simulink model "example_RIEKF"  (R2017b)
settings: Solver=FixedStepDiscrete  StartTime=0.0  StopTime=outputs.messages.Time(end)  RelTol=1e-3  EnableMultiTasking=on
InitFcn:
  | CassieModule.importBuses;
undefined symbols (not defined in the file or in its folder): R0, v0
libraries: lib_StateEstimation x7
settings Model: ParamWorkspaceSource=ReferencedWorkspace  Creator=robot  LastModifiedBy=nboyd
settings DataIOCC: SaveFormat=Array  SaveOutput=off  SignalLogging=off  DSMLogging=off  VisualizeSimOutput=off  SaveTime=off
settings OptimizationCC: DefaultParameterBehavior=Inlined  InlineInvariantSignals=on  LifeSpan=inf  SimCompilerOptimization=on  AccelVerboseBuild=on
settings DebuggingCC: ReadBeforeWriteMsg=DisableAll  WriteAfterWriteMsg=DisableAll  WriteAfterReadMsg=DisableAll  AllowSymbolicDim=off  SFUnexpectedBacktrackingDiag=warning  SFNoUnconditionalDefaultTransitionDiag=warning  SFExecutionAtInitializationDiag=none
settings HardwareCC: ProdBitPerPointer=32  ProdBitPerSizeT=32  ProdBitPerPtrDiffT=32  ProdLargestAtomicFloat=None  ProdWordSize=32  ProdLongLongMode=on  ProdHWDeviceType=Generic->32-bit x86 compatible
settings ModelReferenceCC: UpdateModelReferenceTargets=IfOutOfDate  ParallelModelReferenceMATLABWorkerInit=Copy Base Workspace  ModelReferenceNumInstancesAllowed=Single
settings SFSimCC: SimUserIncludeDirs=gen\kin\src  SFSimEcho=off
settings SFSimCC: SimUserSources=|
  | p_VectorNav_to_RightToeBottom_src.c
  | R_VectorNav_to_RightToeBottom_src.c
  | Jp_VectorNav_to_RightToeBottom_src.c
  | p_VectorNav_to_LeftToeBottom_src.c
  | R_VectorNav_to_LeftToeBottom_src.c
  | Jp_VectorNav_to_LeftToeBottom_src.c
settings RTWCC: SystemTargetFile=slrt.tlc  TLCOptions=-axPCMaxOverloads=1000000000 -axPCMaxOverloadLen=1000000000  TemplateMakefile=slrt_default_tmf  Description=Simulink Real-Time  RTWUseSimCustomCode=on  CustomInclude=gen\kin\src  CodeExecutionProfiling=on  RTWCompilerOptimization=on
settings RTWCC: CustomSource=|
  | p_VectorNav_to_RightToeBottom_src.c
  | R_VectorNav_to_RightToeBottom_src.c
  | Jp_VectorNav_to_RightToeBottom_src.c
  | p_VectorNav_to_LeftToeBottom_src.c
  | R_VectorNav_to_LeftToeBottom_src.c
  | Jp_VectorNav_to_LeftToeBottom_src.c
settings CodeAppCC: GenerateComments=off  MaxIdLength=128  SimulinkBlockComments=off
settings TargetCC: CodeReplacementLibrary=XPC_BLAS  ParMdlRefBuildCompliant=on  ConcurrentExecutionCompliant=on  GeneratePreprocessorConditionals=Use local settings  MatFileLogging=on  MATLABClassNameForMDSCustomization=xpcAperiodicCustomization
settings ConfigComp: CovMetricSettings=dw  CovHtmlReporting=on  CovSaveCumulativeToWorkspaceVar=on  CovSaveSingleToWorkspaceVar=on  CovExternalEMLEnable=off

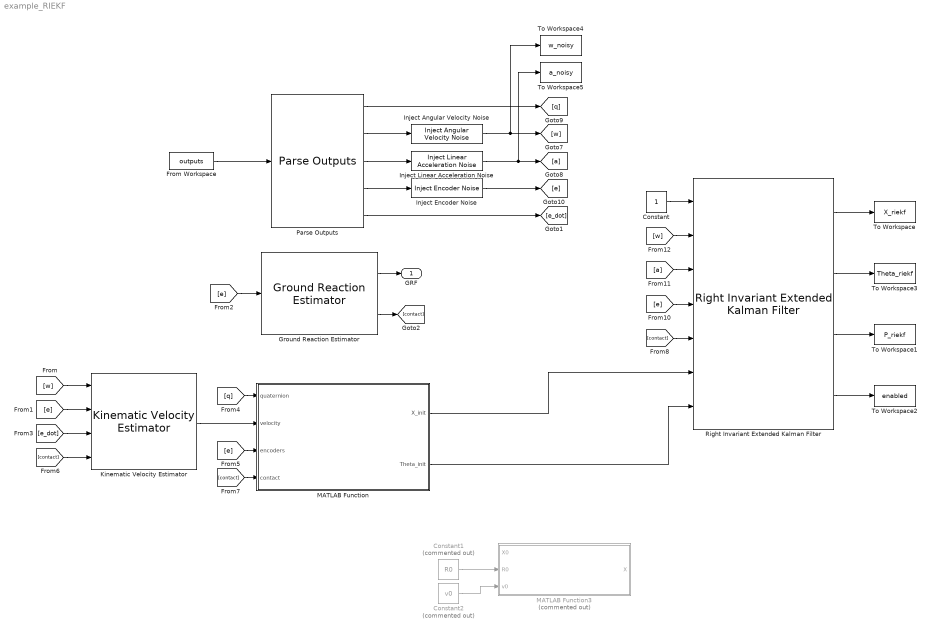
== system example_RIEKF ==
  Constant : Constant  SampleTime=-1
  Constant1 : Constant  Commented=on  Value=R0
  Constant2 : Constant  Commented=on  Value=v0
  From Workspace : FromWorkspace  VariableName=outputs  OutDataTypeStr=Bus: CassieOutBus  Interpolate=off  OutputAfterFinalValue=Holding final value
  Ground Reaction Estimator : lib_StateEstimation/Ground Reaction Estimator
  Inject Angular Velocity Noise : lib_StateEstimation/Inject Angular Velocity Noise
  Inject Encoder Noise : lib_StateEstimation/Inject Encoder Noise
  Inject Linear Acceleration Noise : lib_StateEstimation/Inject Linear Acceleration Noise
  Kinematic Velocity Estimator : lib_StateEstimation/Kinematic Velocity Estimator
  MATLAB Function : MATLAB Function  TreatAsAtomicUnit=on
  MATLAB Function3 : MATLAB Function  Commented=on  TreatAsAtomicUnit=on
  Parse Outputs : lib_StateEstimation/Parse Outputs
  Right Invariant Extended Kalman Filter : lib_StateEstimation/Right Invariant Extended Kalman Filter
  To Workspace : ToWorkspace  VariableName=X_riekf  SaveFormat=Timeseries  SampleTime=-1
  To Workspace1 : ToWorkspace  VariableName=P_riekf  SaveFormat=Timeseries  SampleTime=-1
  To Workspace2 : ToWorkspace  VariableName=enabled  SaveFormat=Timeseries  SampleTime=-1
  To Workspace3 : ToWorkspace  VariableName=Theta_riekf  SaveFormat=Timeseries  SampleTime=-1
  To Workspace4 : ToWorkspace  VariableName=w_noisy  SaveFormat=Timeseries  SampleTime=-1
  To Workspace5 : ToWorkspace  VariableName=a_noisy  SaveFormat=Timeseries  SampleTime=-1
  GRF : Outport
  wires:
  Ground Reaction Estimator/1 -> GRF/1
  [e] -> Ground Reaction Estimator/1
  Parse Outputs/1 -> [q]
  Parse Outputs/2 -> Inject Angular Velocity Noise/1
  Parse Outputs/3 -> Inject Linear Acceleration Noise/1
  Parse Outputs/4 -> Inject Encoder Noise/1
  [w] -> Right Invariant Extended Kalman Filter/2
  [a] -> Right Invariant Extended Kalman Filter/3
  [e] -> Right Invariant Extended Kalman Filter/4
  Right Invariant Extended Kalman Filter/1 -> To Workspace/1
  Right Invariant Extended Kalman Filter/2 -> To Workspace3/1
  Right Invariant Extended Kalman Filter/3 -> To Workspace1/1
  Constant/1 -> Right Invariant Extended Kalman Filter/1
  Parse Outputs/5 -> [e_dot]
  Right Invariant Extended Kalman Filter/4 -> To Workspace2/1
  [w] -> Kinematic Velocity Estimator/1
  [e] -> Kinematic Velocity Estimator/2
  [e_dot] -> Kinematic Velocity Estimator/3
  [q] -> MATLAB Function/1(quaternion)
  Kinematic Velocity Estimator/1 -> MATLAB Function/2(velocity)
  [e] -> MATLAB Function/3(encoders)
  Ground Reaction Estimator/2 -> [contact]
  [contact] -> Kinematic Velocity Estimator/4
  [contact] -> MATLAB Function/4(contact)
  [contact] -> Right Invariant Extended Kalman Filter/5
  MATLAB Function/2(Theta_init) -> Right Invariant Extended Kalman Filter/7
  Constant2/1 -> MATLAB Function3/3(v0)
  Constant1/1 -> MATLAB Function3/2(R0)
  From Workspace/1 -> Parse Outputs/1
  Inject Angular Velocity Noise/1 -> To Workspace4/1, [w]
  Inject Linear Acceleration Noise/1 -> To Workspace5/1, [a]
  Inject Encoder Noise/1 -> [e]
  MATLAB Function/1(X_init) -> Right Invariant Extended Kalman Filter/6

== matlab function example_RIEKF/MATLAB Function ==
  data: quaternion input; velocity input; X_init output; encoders input; contact input; Theta_init output
function [X_init, Theta_init] = InitialStateEstimate(quaternion, velocity, encoders, contact)

R = Angles.Quaternion_to_Rotation(quaternion);
p = zeros(3,1); 
v = R*velocity;
pR = p_VectorNav_to_RightToeBottom(encoders);
pL = p_VectorNav_to_LeftToeBottom(encoders);

if contact(1) == 1
    % Initialize with left foot at 0
    p = -R * pL; % {W}_p_{WL}
elseif contact(2) == 1
    % Initialize with right foot at 0
    p = -R * pR; % {W}_p_{WR}
end

% Initial foot positions
dL = p + R * pL; % {W}_p_{WL}
dR = p + R * pR; % {W}_p_{WR}

% Construct Initial State
X_init = [R, v, p, dL, dR; 0,0,0,1,0,0,0; 0,0,0,0,1,0,0; 0,0,0,0,0,1,0; 0,0,0,0,0,0,1];

Theta_init = zeros(6,1);

end

== matlab function example_RIEKF/MATLAB Function3 ==
  data: X0 input; R0 input; X output; v0 input
function X  = OverwriteState(X0, R0, v0)
X = X0;
X(1:3,1:4) = [R0, v0];
end
